simulink model "pos2airgap"  (R2022b)
settings: Solver=FixedStepAuto  StartTime=0.0  StopTime=10.0  RelTol=1e-3
settings Model: Creator=USUARIO  LastModifiedBy=ramuj

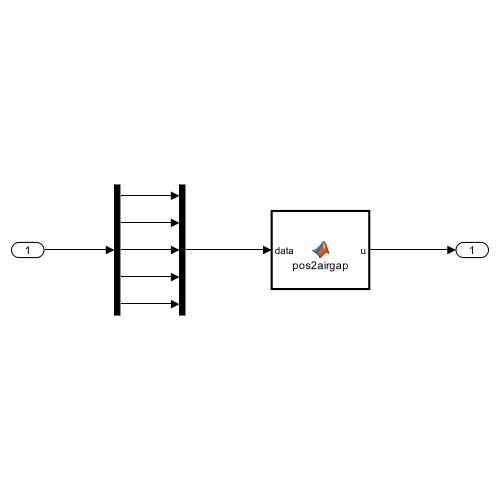
[thumbnail: Simulink's stored preview of the top-level diagram]
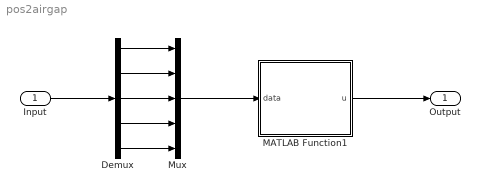
== system pos2airgap ==
  Input : Inport  SampleTime=1/7500
  Demux : Demux  Outputs=5
  MATLAB Function1 : MATLAB Function  TreatAsAtomicUnit=on
  Mux : Mux  Inputs=5
  Output : Outport
  wires:
  MATLAB Function1/1(u) -> Output/1
  Demux/4 -> Mux/4
  Demux/1 -> Mux/1
  Mux/1 -> MATLAB Function1/1(data)
  Input/1 -> Demux/1
  Demux/2 -> Mux/2
  Demux/3 -> Mux/3
  Demux/5 -> Mux/5

== matlab function pos2airgap/MATLAB Function1 ==
  data: data input; u output
function u = pos2airgap(data)

% CONSTANTES
x_sragy = 0.7681;
y_sragy = 0.0951;
z_sragy = 0.07922;
x_sragz = 0.76785;
y_sragz = 0.22269;
z_sragz = -0.09493;
z_infr = 0.6328;
grosorz = 0.015;
grosory = 0.005;

y = data(1);
z = data(2);
rotx = data(3);
roty = data(4);
rotz = data(5);

% DISTANCIAS
airgap5 = + y + y_sragy * cos(rotz) + x_sragy * sin(rotz) - z_sragy * sin(rotx) - grosory;
airgap6 = - y + y_sragy * cos(rotz) - x_sragy * sin(rotz) + z_sragy * sin(rotx) - grosory;
airgap7 = + y + y_sragy * cos(rotz) - x_sragy * sin(rotz) - z_sragy * sin(rotx) - grosory;
airgap8 = - y + y_sragy * cos(rotz) + x_sragy * sin(rotz) + z_sragy * sin(rotx) - grosory;

airgap1 =  -z  + z_infr  - z_sragz * cos(roty) + x_sragz * sin(roty) - y_sragz * sin(rotx);
airgap2 =  -z  + z_infr  - z_sragz * cos(roty) + x_sragz * sin(roty) + y_sragz * sin(rotx);
airgap3 =  -z  + z_infr  - z_sragz * cos(roty) - x_sragz * sin(roty) - y_sragz * sin(rotx);
airgap4 =  -z  + z_infr  - z_sragz * cos(roty) - x_sragz * sin(roty) + y_sragz * sin(rotx);

u =[airgap1, airgap2, airgap3, airgap4, airgap5, airgap6, airgap7, airgap8]';
